simulink model "Sinusoidal_tracking_P3"  (R2022a)
settings: Solver=ode45  StartTime=0.0  StopTime=100  RelTol=1e-3
values from neighbouring files (symbols this model uses):
  absolute_encoder_counts_per_revolution = 128    [ELEN90064_Project_Parameters.m]
  C = [0 1 0 0 0]    [DesignProjectP2.m]    (also in DesignProjectP3.m = [1 0 0 0 0; DesignProject_OffsetP3.m = [1 0 0 0 0; mpc_example_regulation.m = [1 0 0 0 0; mpc_example_tracking.m = [1 0 0 0 0)
  C_d2 = [1 0]    [DesignProjectP3.m]    (also in DesignProject_OffsetP3.m)
  D_sin = c2d(G_sin, T, 'zoh')    [DesignProjectP3.m]    (also in DesignProject_OffsetP3.m)
  Dp = c2d(Gp, T, 'zoh')    [DesignProjectP3.m]    (also in DesignProject_OffsetP3.m; mpc_example_regulation.m; mpc_example_tracking.m)
  gyro_sigma_drift = deg2rad(5)    [ELEN90064_Project_Parameters.m]
  init = [theta_m_init; theta_l_init; thetadot_m_init; thetadot_l_init; Ia_init]    [ELEN90064_Project_Parameters.m]
  K = K(2:6)    [DesignProjectP2.m]    (also in DesignProjectP3.m = K_dist(1:5); DesignProject_OffsetP3.m = K_dist(2:6); phase2_emc.m = place(A,B,desired_poles))
  K_d = K_dist(8:9)    [DesignProjectP3.m]    (also in DesignProject_OffsetP3.m = K_dist(9:10))
  K_sin = K_dist(6:7)    [DesignProjectP3.m]    (also in DesignProject_OffsetP3.m = K_dist(7:8))
  L_disc = L_disct'    [DesignProjectP3.m]    (also in DesignProject_OffsetP3.m; mpc_example_regulation.m; mpc_example_tracking.m)
  w = 2*pi*1/4    (= 1.57079632679)    [DesignProjectP3.m]    (also in DesignProject_OffsetP3.m)
settings Model: Creator=Admin  LastModifiedBy=Admin

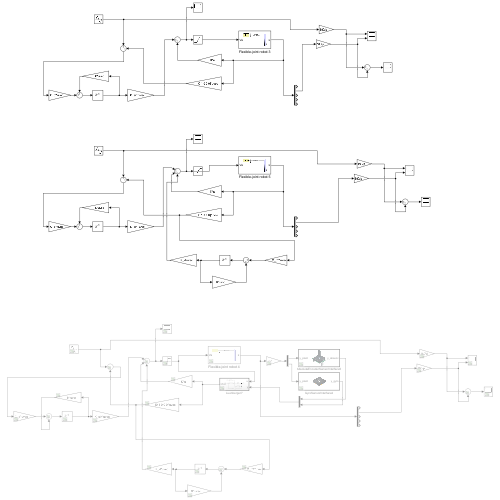
[thumbnail: Simulink's stored preview of the top-level diagram]
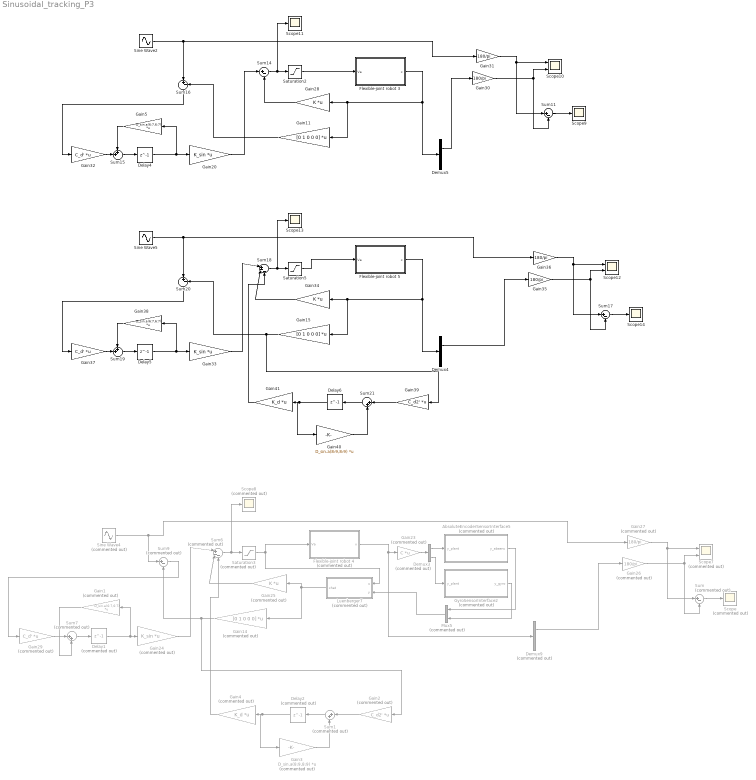
== system Sinusoidal_tracking_P3 ==
  AbsoluteEncoderSensorInterface5 : Subsystem  Commented=on  TreatAsAtomicUnit=on
      mask Display: image('$imagefile'); % Use "Edit Image" on toolstrip to change.
  Delay1 : Delay  Commented=on  DelayLength=1
  Delay2 : Delay  Commented=on  DelayLength=1
  Delay4 : Delay  DelayLength=1
  Delay5 : Delay  DelayLength=1
  Delay6 : Delay  DelayLength=1
  Demux3 : Demux  Commented=on  Outputs=2
  Demux4 : Demux  Outputs=5
  Demux5 : Demux  Outputs=5
  Demux9 : Demux  Commented=on  Outputs=5
  Flexible-joint robot 3 : Subsystem
      mask Display: image('$imagefile'); % Use "Edit Image" on toolstrip to change.
  Flexible-joint robot 4 : Subsystem  Commented=on
      mask Display: image('$imagefile'); % Use "Edit Image" on toolstrip to change.
  Flexible-joint robot 5 : Subsystem
      mask Display: image('$imagefile'); % Use "Edit Image" on toolstrip to change.
  Gain1 : Gain  Commented=on  Gain=D_sin.a(6:7,6:7)  Multiplication=Matrix(K*u) (u vector)
  Gain11 : Gain  Gain=[0 1 0 0 0]  Multiplication=Matrix(K*u) (u vector)
  Gain14 : Gain  Commented=on  Gain=[0 1 0 0 0]  Multiplication=Matrix(K*u) (u vector)
  Gain15 : Gain  Gain=[0 1 0 0 0]  Multiplication=Matrix(K*u) (u vector)
  Gain2 : Gain  Commented=on  Gain=C_d2'  Multiplication=Matrix(K*u) (u vector)
  Gain20 : Gain  Gain=K_sin  Multiplication=Matrix(K*u) (u vector)
  Gain23 : Gain  Commented=on  Gain=C  Multiplication=Matrix(K*u)
  Gain24 : Gain  Commented=on  Gain=K_sin  Multiplication=Matrix(K*u) (u vector)
  Gain25 : Gain  Commented=on  Gain=K  Multiplication=Matrix(K*u)
  Gain26 : Gain  Commented=on  Gain=180/pi
  Gain27 : Gain  Commented=on  Gain=180/pi
  Gain28 : Gain  Gain=K  Multiplication=Matrix(K*u)
  Gain29 : Gain  Commented=on  Gain=C_d'  Multiplication=Matrix(K*u) (u vector)
  Gain3 : Gain  Commented=on  Gain=D_sin.a(8:9,8:9)  Multiplication=Matrix(K*u) (u vector)
  Gain{30..31,35..36} (4 alike) : Gain  Gain=180/pi
  Gain32 : Gain  Gain=C_d'  Multiplication=Matrix(K*u) (u vector)
  Gain33 : Gain  Gain=K_sin  Multiplication=Matrix(K*u) (u vector)
  Gain34 : Gain  Gain=K  Multiplication=Matrix(K*u)
  Gain37 : Gain  Gain=C_d'  Multiplication=Matrix(K*u) (u vector)
  Gain38 : Gain  Gain=D_sin.a(6:7,6:7)  Multiplication=Matrix(K*u) (u vector)
  Gain39 : Gain  Gain=C_d2'  Multiplication=Matrix(K*u) (u vector)
  Gain4 : Gain  Commented=on  Gain=K_d  Multiplication=Matrix(K*u) (u vector)
  Gain40 : Gain  Gain=D_sin.a(8:9,8:9)  Multiplication=Matrix(K*u) (u vector)
  Gain41 : Gain  Gain=K_d  Multiplication=Matrix(K*u) (u vector)
  Gain5 : Gain  Gain=D_sin.a(6:7,6:7)  Multiplication=Matrix(K*u) (u vector)
  GyroSensorInterface2 : Subsystem  Commented=on  TreatAsAtomicUnit=on
      mask Display: image('$imagefile'); % Use "Edit Image" on toolstrip to change.
  Luenberger7 : Subsystem  Commented=on  TreatAsAtomicUnit=on
  Mux5 : Mux  Commented=on  Inputs=2
  Saturation2 : Saturate  UpperLimit=6  LowerLimit=-6
  Saturation3 : Saturate  Commented=on  UpperLimit=6  LowerLimit=-6
  Saturation5 : Saturate  UpperLimit=6  LowerLimit=-6
  Scope : Scope  Commented=on
  Scope10 : Scope  NumInputPorts=2
  Scope{9,11,13..14} (4 alike) : Scope
  Scope12 : Scope  NumInputPorts=2
  Scope7 : Scope  Commented=on  NumInputPorts=2
  Scope8 : Scope  Commented=on
  Sine Wave2 : Sin  Amplitude=deg2rad(30)  Frequency=w  Phase=deg2rad(30)  SampleTime=0
  Sine Wave4 : Sin  Commented=on  Amplitude=deg2rad(30)  Frequency=w  Phase=deg2rad(30)  SampleTime=0
  Sine Wave5 : Sin  Amplitude=deg2rad(30)  Frequency=w  Phase=deg2rad(30)  SampleTime=0
  Sum : Sum  Commented=on  Inputs=|+-
  Sum1 : Sum  Commented=on  Inputs=|++
  Sum{11,14,16..17,20} (5 alike) : Sum  Inputs=|+-
  Sum15 : Sum  Inputs=++|
  Sum18 : Sum  Inputs=|+--
  Sum19 : Sum  Inputs=++|
  Sum21 : Sum  Inputs=|++
  Sum6 : Sum  Commented=on  Inputs=|+--
  Sum7 : Sum  Commented=on  Inputs=|++
  Sum9 : Sum  Commented=on  Inputs=|+-
  wires:
  GyroSensorInterface2/1(y_gyro) -> Mux5/2
  AbsoluteEncoderSensorInterface5/1(y_absenc) -> Mux5/1
  Demux3/1 -> AbsoluteEncoderSensorInterface5/1(y_plant)
  Sum9/1 -> Gain29/1
  Delay1/1 -> Gain1/1, Gain24/1
  Gain24/1 -> Sum6/1
  Gain1/1 -> Sum7/2
  Sum6/1 -> Scope8/1, Saturation3/1
  Gain29/1 -> Sum7/1
  Sum7/1 -> Delay1/1
  Demux3/2 -> GyroSensorInterface2/1(y_plant)
  Luenberger7/1(xhat) -> Gain25/1, Gain14/1
  Gain25/1 -> Sum6/2
  Gain26/1 -> Sum/2, Scope7/2
  Flexible-joint robot 4/1(x) -> Gain23/1, Demux9/1
  Gain27/1 -> Sum/1, Scope7/1
  Sine Wave4/1 -> Gain27/1, Sum9/1
  Mux5/1 -> Luenberger7/2(y)
  Saturation3/1 -> Luenberger7/1(u), Flexible-joint robot 4/1(Va)
  Demux9/2 -> Gain26/1
  Gain23/1 -> Demux3/1
  Sum/1 -> Scope/1
  Sum11/1 -> Scope9/1
  Demux5/2 -> Gain30/1
  Saturation2/1 -> Flexible-joint robot 3/1(Va)
  Sine Wave2/1 -> Gain31/1, Sum16/1
  Gain31/1 -> Scope10/1, Sum11/1
  Gain30/1 -> Scope10/2, Sum11/2
  Gain28/1 -> Sum14/2
  Flexible-joint robot 3/1(x) -> Gain11/1, Gain28/1, Demux5/1
  Sum15/1 -> Delay4/1
  Gain32/1 -> Sum15/2
  Sum14/1 -> Saturation2/1, Scope11/1
  Gain5/1 -> Sum15/1
  Gain20/1 -> Sum14/1
  Delay4/1 -> Gain20/1, Gain5/1
  Gain11/1 -> Sum16/2
  Sum16/1 -> Gain32/1
  Sum20/1 -> Gain37/1
  Delay5/1 -> Gain38/1, Gain33/1
  Gain33/1 -> Sum18/1
  Gain38/1 -> Sum19/1
  Sum18/1 -> Scope13/1, Saturation5/1
  Gain37/1 -> Sum19/2
  Sum19/1 -> Delay5/1
  Flexible-joint robot 5/1(x) -> Demux4/1, Gain34/1, Gain15/1
  Gain34/1 -> Sum18/2
  Gain35/1 -> Sum17/2, Scope12/2
  Gain36/1 -> Sum17/1, Scope12/1
  Sine Wave5/1 -> Sum20/1, Gain36/1
  Saturation5/1 -> Flexible-joint robot 5/1(Va)
  Demux4/2 -> Gain35/1
  Sum17/1 -> Scope14/1
  Delay6/1 -> Gain41/1, Gain40/1
  Gain40/1 -> Sum21/2
  Sum21/1 -> Delay6/1
  Gain39/1 -> Sum21/1
  Gain15/1 -> Gain39/1, Sum20/2
  Gain41/1 -> Sum18/3
  Gain4/1 -> Sum6/3
  Gain14/1 -> Gain2/1, Sum9/2
  Gain2/1 -> Sum1/1
  Sum1/1 -> Delay2/1
  Gain3/1 -> Sum1/2
  Delay2/1 -> Gain3/1, Gain4/1

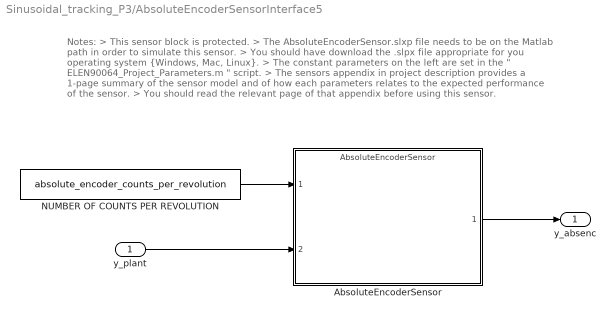
== system Sinusoidal_tracking_P3/AbsoluteEncoderSensorInterface5 ==
  note: Notes:
      | > This sensor block is protected.
      | > The AbsoluteEncoderSensor.slxp file needs to be on the Matlab path in order to simulate this sensor.
      | > You should have download the .slpx file appropriate for you operating system {Windows, Mac, Linux}.
      | > The constant parameters on the left are set in the " ELEN90064_Project_Parameters.m " script.
      | > The sensors appendix in project description provides a 1-page summary of the sensor model and of how each parameters relates to the expected performance of the sensor.
      | > You should read the relevant page of that appendix before using this sensor.
  y_plant : Inport
  AbsoluteEncoderSensor : ModelReference  ModelNameDialog=AbsoluteEncoderSensor.slxp  ModelReferenceVersion=1.16  CopyOfModelProtected=on
  NUMBER OF COUNTS PER REVOLUTION : Constant  Value=absolute_encoder_counts_per_revolution
  y_absenc : Outport
  wires:
  NUMBER OF COUNTS PER REVOLUTION/1 -> AbsoluteEncoderSensor/1
  y_plant/1 -> AbsoluteEncoderSensor/2
  AbsoluteEncoderSensor/1 -> y_absenc/1

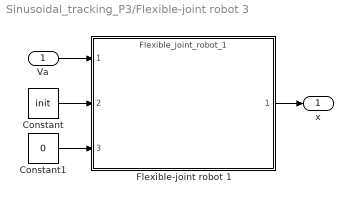
== system Sinusoidal_tracking_P3/Flexible-joint robot 3 ==
  Va : Inport
  Constant : Constant  Value=init
  Constant1 : Constant  Value=0
  Flexible-joint robot 1 : ModelReference  ModelNameDialog=Flexible_joint_robot_1  ModelReferenceVersion=1.65  CopyOfModelProtected=on
  x : Outport
  wires:
  Constant/1 -> Flexible-joint robot 1/2
  Flexible-joint robot 1/1 -> x/1
  Va/1 -> Flexible-joint robot 1/1
  Constant1/1 -> Flexible-joint robot 1/3

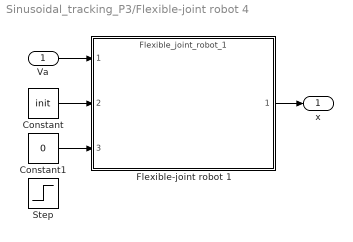
== system Sinusoidal_tracking_P3/Flexible-joint robot 4 ==
  Va : Inport
  Constant : Constant  Value=init
  Constant1 : Constant  Value=0
  Flexible-joint robot 1 : ModelReference  ModelNameDialog=Flexible_joint_robot_1  ModelReferenceVersion=1.65  CopyOfModelProtected=on
  Step : Step  After=0.05  SampleTime=0
  x : Outport
  wires:
  Constant1/1 -> Flexible-joint robot 1/3
  Va/1 -> Flexible-joint robot 1/1
  Flexible-joint robot 1/1 -> x/1
  Constant/1 -> Flexible-joint robot 1/2

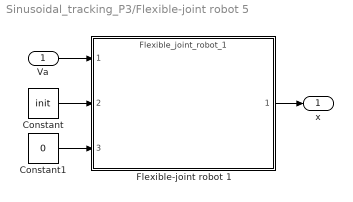
== system Sinusoidal_tracking_P3/Flexible-joint robot 5 ==
  Va : Inport
  Constant : Constant  Value=init
  Constant1 : Constant  Value=0
  Flexible-joint robot 1 : ModelReference  ModelNameDialog=Flexible_joint_robot_1  ModelReferenceVersion=1.65  CopyOfModelProtected=on
  x : Outport
  wires:
  Constant1/1 -> Flexible-joint robot 1/3
  Va/1 -> Flexible-joint robot 1/1
  Flexible-joint robot 1/1 -> x/1
  Constant/1 -> Flexible-joint robot 1/2

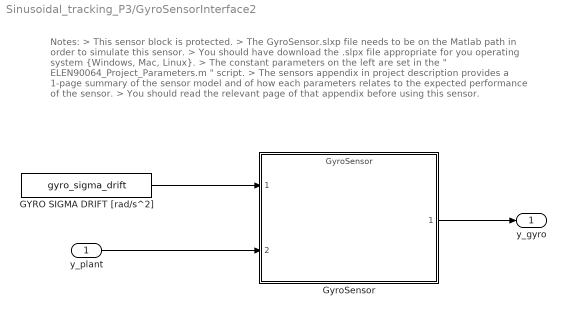
== system Sinusoidal_tracking_P3/GyroSensorInterface2 ==
  note: Notes:
      | > This sensor block is protected.
      | > The GyroSensor.slxp file needs to be on the Matlab path in order to simulate this sensor.
      | > You should have download the .slpx file appropriate for you operating system {Windows, Mac, Linux}.
      | > The constant parameters on the left are set in the " ELEN90064_Project_Parameters.m " script.
      | > The sensors appendix in project description provides a 1-page summary of the sensor model and of how each parameters relates to the expected performance of the sensor.
      | > You should read the relevant page of that appendix before using this sensor.
  y_plant : Inport
  GYRO SIGMA DRIFT [rad/s^2] : Constant  Value=gyro_sigma_drift
  GyroSensor : ModelReference  ModelNameDialog=GyroSensor.slxp  ModelReferenceVersion=1.18  CopyOfModelProtected=on
  y_gyro : Outport
  wires:
  GYRO SIGMA DRIFT [rad/s^2]/1 -> GyroSensor/1
  y_plant/1 -> GyroSensor/2
  GyroSensor/1 -> y_gyro/1

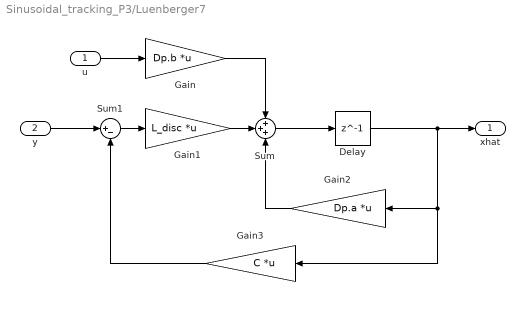
== system Sinusoidal_tracking_P3/Luenberger7 ==
  u : Inport
  y : Inport  Port=2
  Delay : Delay  DelayLength=1
  Gain : Gain  Gain=Dp.b  Multiplication=Matrix(K*u) (u vector)
  Gain1 : Gain  Gain=L_disc  Multiplication=Matrix(K*u) (u vector)
  Gain2 : Gain  Gain=Dp.a  Multiplication=Matrix(K*u) (u vector)
  Gain3 : Gain  Gain=C  Multiplication=Matrix(K*u) (u vector)
  Sum : Sum  Inputs=+++
  Sum1 : Sum  Inputs=|+-
  xhat : Outport
  wires:
  u/1 -> Gain/1
  Gain/1 -> Sum/1
  y/1 -> Sum1/1
  Sum1/1 -> Gain1/1
  Gain1/1 -> Sum/2
  Sum/1 -> Delay/1
  Delay/1 -> Gain3/1, Gain2/1, xhat/1
  Gain2/1 -> Sum/3
  Gain3/1 -> Sum1/2
